simulink model "verAmotor_control"  (R2016a)
settings: Solver=FixedStepDiscrete  StartTime=0.0  StopTime=5  FixedStep=1e-3  RelTol=1e-3
PostLoadFcn:
  | J=3.2284e-6
  | b=3.5066e-6
  | K=0.0274
  | R=4
  | L=2.75e-6
libraries: simulink x1
settings Model: Creator=maen  LastModifiedBy=andrea
settings DataIOCC: LimitDataPoints=on  SaveFormat=Array  SignalLoggingSaveFormat=ModelDataLogs
settings OptimizationCC: ExpressionDepthLimit=2147483647
settings DebuggingCC: UnderspecifiedInitializationDetection=Classic  MergeDetectMultiDrivingBlocksExec=none  SolverPrmCheckMsg=warning  FcnCallInpInsideContextMsg=EnableAllAsWarning  StateNameClashWarn=warning
settings HardwareCC: ProdBitPerPointer=32  ProdLargestAtomicFloat=None  ProdIntDivRoundTo=Undefined  ProdEndianess=Unspecified  ProdWordSize=32  ProdHWDeviceType=32-bit Generic
settings ModelReferenceCC: PropagateSignalLabelsOutOfModel=off
settings GRTTargetCC: CombineOutputUpdateFcns=off  GRTInterface=on

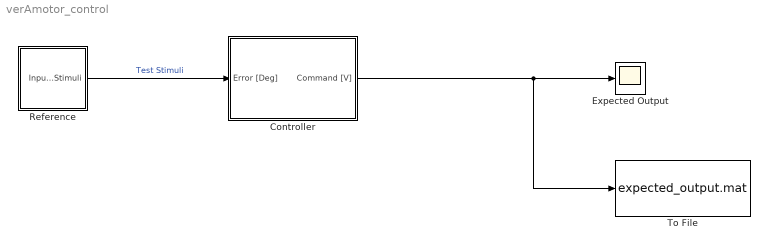
== system verAmotor_control ==
  Controller : Subsystem
  "Expected Output " : Scope
  Reference : Subsystem
  To File : ToFile  Filename=expected_output.mat
  wires:
  Controller/1(Command [V]) -> To File/1, "Expected Output "/1
  Reference/1(Input Stimuli) -> Controller/1(Error [Deg])  "Test Stimuli"

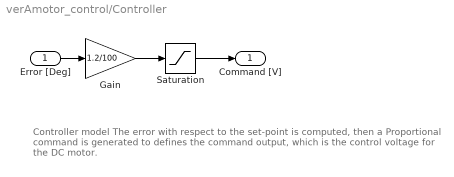
== system verAmotor_control/Controller ==
  note: Controller model
      | The error with respect to the set-point is computed, then a Proportional command
      | is generated to defines the command output, which is the control voltage for the DC motor.
  Error [Deg] : Inport
  Gain : Gain  Gain=1.2/100
  Saturation : Saturate  UpperLimit=1  LowerLimit=-1
  Command [V] : Outport
  wires:
  Gain/1 -> Saturation/1
  Error [Deg]/1 -> Gain/1
  Saturation/1 -> Command [V]/1

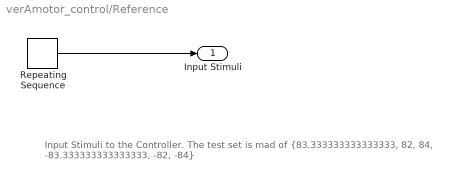
== system verAmotor_control/Reference ==
  note: Input Stimuli to the Controller. The test set is mad of {83.333333333333333, 82, 84, -83.333333333333333, -82, -84}
  Repeating Sequence : simulink/Sources/Repeating Sequence  rep_seq_t=[0 1 2 3 4 5]  rep_seq_y=[83.333333333333333 82 84 -83.333333333333333 -82 -84].'
  Input Stimuli : Outport
  wires:
  Repeating Sequence/1 -> Input Stimuli/1
